simulink model "simpleTreeDiff"  (R2023b)
settings: Solver=VariableStepAuto  StartTime=0.0  StopTime=10.0  RelTol=1e-3
settings Model: Creator=neham  LastModifiedBy=neham

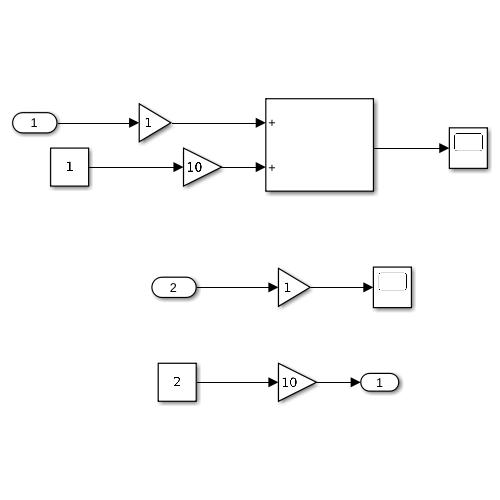
[thumbnail: Simulink's stored preview of the top-level diagram]
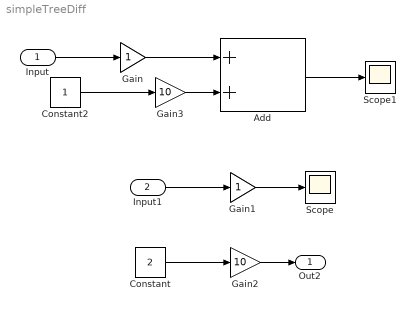
== system simpleTreeDiff ==
  Input : Inport
  Input1 : Inport  Port=2
  Add : Sum
  Constant : Constant  Value=2
  Constant2 : Constant
  Gain : Gain
  Gain1 : Gain
  Gain2 : Gain  Gain=10
  Gain3 : Gain  Gain=10
  Scope : Scope
  Scope1 : Scope
  Out2 : Outport
  wires:
  Input/1 -> Gain/1
  Gain/1 -> Add/1
  Add/1 -> Scope1/1
  Constant/1 -> Gain2/1
  Input1/1 -> Gain1/1
  Gain1/1 -> Scope/1
  Gain2/1 -> Out2/1
  Constant2/1 -> Gain3/1
  Gain3/1 -> Add/2
